simulink model "ModelloTeam1Test"  (R2022b)
settings: Solver=FixedStepAuto  StartTime=0.0  StopTime=2500  RelTol=1e-3  EnableMultiTasking=on
libraries: mbedblockslib x7
settings Model: ExtModeTrigDuration=10  Creator=giova  LastModifiedBy=giova
settings OptimizationCC: EnhancedBackFolding=on  PassReuseOutputArgsAs=Individual arguments  ZeroExternalMemoryAtStartup=off  ZeroInternalMemoryAtStartup=off  MaxStackSize=64  OptimizeBlockOrder=speed  DifferentSizesBufferReuse=on  OptimizationCustomize=off  EfficientTunableParamExpr=on
settings DebuggingCC: InheritedTsInSrcMsg=error  ParameterTunabilityLossMsg=error
settings HardwareCC: ProdBitPerPointer=32  ProdBitPerSizeT=32  ProdBitPerPtrDiffT=32  ProdLargestAtomicInteger=Long  ProdLargestAtomicFloat=Double  ProdWordSize=32  ProdLongLongMode=on  ProdHWDeviceType=ARM Compatible->ARM Cortex  UseEmbeddedCoderFeatures=off
settings SFSimCC: MATLABDynamicMemAlloc=off
settings RTWCC: Description=Embedded Coder  SystemTargetFile=ert.tlc  HardwareBoard=STM32 Nucleo F401RE  TLCOptions=-aInlineSetEventsForThisBaseRateFcn=TLC_FALSE -aSuppressMultiTaskScheduler=TLC_FALSE -aRateBasedStepFcn=1  TemplateMakefile=ert_default_tmf  Toolchain=GNU Tools for ARM Embedded Processors
settings CodeAppCC: ForceParamTrailComments=on  IgnoreCustomStorageClasses=off  OperatorAnnotations=on  SimulinkDataObjDesc=on  SFDataObjDesc=on  InsertBlockDesc=on
settings ERTTargetCC: SupportNonInlinedSFcns=on  ExtModeTransport=3  ExtModeStaticAlloc=on  ExtModeStaticAllocSize=2000  ExtModeMexFile=ext_xcp  ExtModeIntrfLevel=Level2 - Open

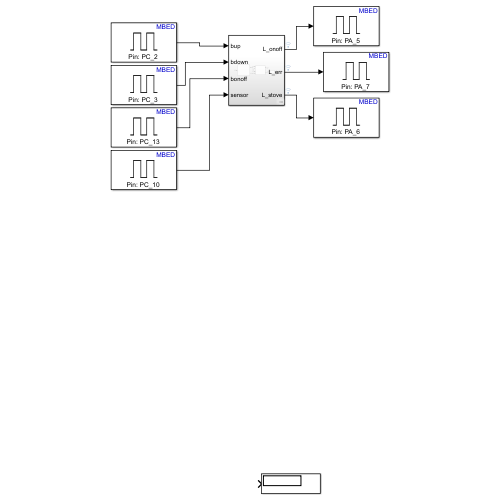
[thumbnail: Simulink's stored preview of the top-level diagram]
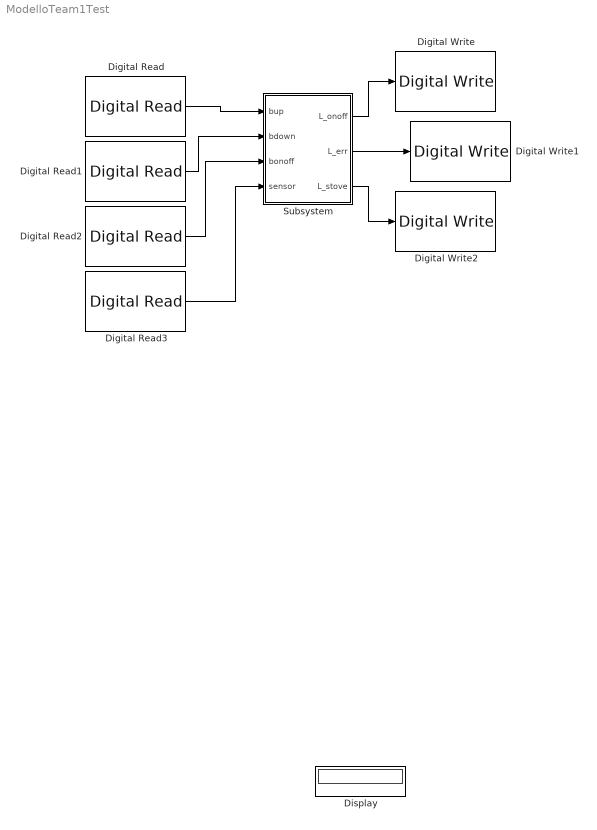
== system ModelloTeam1Test ==
  Digital Read : mbedblockslib/Digital Read  Pin=PC_2  Direction=input  SampleTime=-1
      settings: LibrarySourceBlock=stmnucleorootlib/Common/Digital Read
  Digital Read1 : mbedblockslib/Digital Read  Pin=PC_3  Direction=input  SampleTime=-1
      settings: LibrarySourceBlock=stmnucleorootlib/Common/Digital Read
  Digital Read2 : mbedblockslib/Digital Read  Pin=PC_13  Direction=input  SampleTime=-1
      settings: LibrarySourceBlock=stmnucleorootlib/Common/Digital Read
  Digital Read3 : mbedblockslib/Digital Read  Pin=PC_10  Direction=input  SampleTime=-1
      settings: LibrarySourceBlock=stmnucleorootlib/Common/Digital Read
  Digital Write : mbedblockslib/Digital Write  Pin=PA_5  Direction=output
      settings: LibrarySourceBlock=stmnucleorootlib/Common/Digital Write
  Digital Write1 : mbedblockslib/Digital Write  Pin=PA_7  Direction=output
      settings: LibrarySourceBlock=stmnucleorootlib/Common/Digital Write
  Digital Write2 : mbedblockslib/Digital Write  Pin=PA_6  Direction=output
      settings: LibrarySourceBlock=stmnucleorootlib/Common/Digital Write
  Display : Display
  Subsystem : Subsystem
  wires:
  Digital Read/1 -> Subsystem/1(bup)
  Digital Read1/1 -> Subsystem/2(bdown)
  Digital Read2/1 -> Subsystem/3(bonoff)
  Digital Read3/1 -> Subsystem/4(sensor)
  Subsystem/1(L_onoff) -> Digital Write/1
  Subsystem/2(L_err) -> Digital Write1/1
  Subsystem/3(L_stove) -> Digital Write2/1

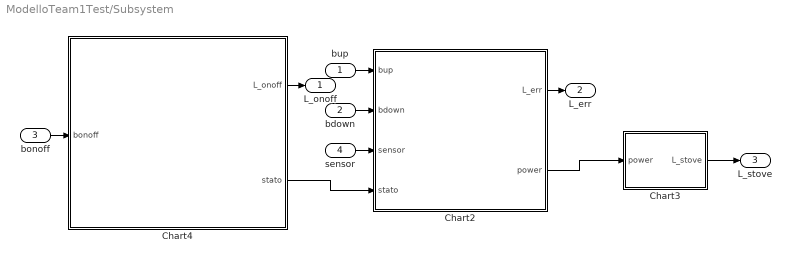
== system ModelloTeam1Test/Subsystem ==
  bup : Inport
  bdown : Inport  Port=2
  bonoff : Inport  Port=3
  sensor : Inport  Port=4
  Chart2 : Stateflow chart  TreatAsAtomicUnit=on
  Chart3 : Stateflow chart  TreatAsAtomicUnit=on
  Chart4 : Stateflow chart  TreatAsAtomicUnit=on
  L_onoff : Outport
  L_err : Outport  Port=2
  L_stove : Outport  Port=3
  wires:
  bdown/1 -> Chart2/2(bdown)
  bup/1 -> Chart2/1(bup)
  Chart2/2(power) -> Chart3/1(power)
  Chart3/1(L_stove) -> L_stove/1
  sensor/1 -> Chart2/3(sensor)
  Chart2/1(L_err) -> L_err/1
  bonoff/1 -> Chart4/1(bonoff)
  Chart4/1(L_onoff) -> L_onoff/1
  Chart4/2(stato) -> Chart2/4(stato)

== stateflow chart ModelloTeam1Test/Subsystem/Chart3 ==
  settings: updateMethod=DISCRETE  sampleTime=0.25
  state Stove_management
    state Blinking_stove
      state Led_on
        en: L_stove=ON;
      state Led_off
        en: L_stove = OFF;
      (default) -> Led_on
      Led_off -> Led_on : after(power,sec)
      Led_on -> Led_off : after(power,sec)
    state Starting_power
      en: L_stove=OFF;
    (default) -> Starting_power
    Blinking_stove -> Starting_power : [power==MAX_TIMING]
    Starting_power -> Blinking_stove : [power<MAX_TIMING]
  data: ON local =true; OFF local =false; L_stove output; power input; MAX_TIMING local =4

== stateflow chart ModelloTeam1Test/Subsystem/Chart2 ==
  settings: updateMethod=DISCRETE  sampleTime=0.25
  state Power_and_error_management
    state Power_management [parallel]
      settings: executionOrder=1
      state PowerUD_manager_on
        state PowerUp
          en: temp_power=temp_power/2
        state Check_buttons
          en: power=temp_power;
        state PowerDown
          en: temp_power=temp_power*2
        PowerUp -> Check_buttons [order 4] : [power==MAX_TIMING & sensor~=ACTIVE]{temp_power=MAX_TIMING}
        PowerUp -> Check_buttons [order 2] : after(TIMER,sec)
        Check_buttons -> PowerUp [order 1] : [power~=MIN_TIMING  & bup_second==PRESSED]
        PowerUp -> PowerUp [order 3] : [temp_power~=MIN_TIMING  & bup_second==PRESSED]
        PowerUp -> PowerDown [order 1] : [bdown_second==PRESSED]
        PowerDown -> PowerUp [order 1] : [ bup_second==PRESSED]
        (default) -> Check_buttons
        Check_buttons -> PowerDown [order 2] : [power~=MAX_TIMING & bdown_second==PRESSED]
        PowerDown -> Check_buttons [order 4] : [power==MAX_TIMING & sensor~=ACTIVE]{temp_power=MAX_TIMING}
        PowerDown -> Check_buttons [order 2] : after(TIMER,sec)
        PowerDown -> PowerDown [order 3] : [temp_power~=MAX_TIMING & bdown_second==PRESSED]
      state PowerUD_manager_off
        en: temp_power=MAX_TIMING
        power=MAX_TIMING;
      (default) -> PowerUD_manager_off
      PowerUD_manager_off -> PowerUD_manager_on : [stato==ON]
      PowerUD_manager_on -> PowerUD_manager_off : [stato==OFF]
    state Button_up_down_management [parallel]
      settings: executionOrder=2
      state Button_up_down_manager_on
        state Longpressed_DOWN_button
          en: bdown_second = RELEASED;
        state Longpressed_UP_botton
          en: bup_second = RELEASED;
        state Pressed_DOWN_button
          en: bdown_second = RELEASED;
          on after(BUTTONDURATION,sec):
          bdown_second=PRESSED;
        state Pressed_UP_botton
          en: bup_second = RELEASED;
          on after(BUTTONDURATION,sec):
          bup_second=PRESSED;
        state Wait_Up_Down_button
          en: bup_second=RELEASED;
          bdown_second=RELEASED;
        Longpressed_UP_botton -> Wait_Up_Down_button : [bup==RELEASED]
        Pressed_UP_botton -> Longpressed_UP_botton [order 2] : [bup_second==PRESSED & bup == PRESSED]
        Pressed_DOWN_button -> Longpressed_DOWN_button [order 1] : [bdown_second==PRESSED & bdown == PRESSED]
        Longpressed_DOWN_button -> Wait_Up_Down_button : [bdown==RELEASED]
        Pressed_UP_botton -> Wait_Up_Down_button [order 1] : [bup==RELEASED | sensor ~=ACTIVE]
        Pressed_DOWN_button -> Wait_Up_Down_button [order 2] : [bdown==RELEASED | sensor~=ACTIVE]
        Wait_Up_Down_button -> Pressed_UP_botton [order 2] : [bup==PRESSED & sensor==ACTIVE]
        (default) -> Wait_Up_Down_button
        Wait_Up_Down_button -> Pressed_DOWN_button [order 1] : [bdown==PRESSED & sensor==ACTIVE]
      state Button_up_down_manager_off
      Button_up_down_manager_off -> Button_up_down_manager_on : [stato==ON]
      Button_up_down_manager_on -> Button_up_down_manager_off : [stato==OFF]
      (default) -> Button_up_down_manager_off
    state Error_management [parallel]
      settings: executionOrder=3
      state Error_manager_on
        state Wait_blinking
          en: power=MAX_TIMING;
          temp_power=MAX_TIMING;
        state Check_error
        state Start_error
          en: L_err=ON;
          ex: L_err =OFF;
        (default) -> Wait_blinking
        Check_error -> Wait_blinking [order 2] : [power==MAX_TIMING]
        Wait_blinking -> Check_error : [power<MAX_TIMING]
        Start_error -> Check_error [order 1] : [sensor==ACTIVE]
        Check_error -> Start_error [order 1] : [sensor~=ACTIVE]
        Start_error -> Wait_blinking [order 2] : after(ERR_TIMER,sec)
      state Error_manager_off
        en: L_err=OFF;
      Error_manager_off -> Error_manager_on : [stato==ON]
      (default) -> Error_manager_off
      Error_manager_on -> Error_manager_off : [stato==OFF]
  (default) -> Power_and_error_management
  data: bup input; bdown input; sensor input; L_err output; RELEASED local =true; PRESSED local =false; BUTTONDURATION local =1; bup_second local; bdown_second local; ACTIVE local =0; ERR_TIMER local =10; ON local =true; OFF local =false; TIMER local =5; temp_power local; power output; stato input boolean; MAX_TIMING local =4; MIN_TIMING local =0.25

== stateflow chart ModelloTeam1Test/Subsystem/Chart4 ==
  settings: updateMethod=DISCRETE  sampleTime=0.25
  state PowerOFF_management
    state PowerOFF_manager_on
      state Pressed_OFF_button
        en: bonoff_second = RELEASED;
        on after(BUTTONDURATION,sec):
        bonoff_second=PRESSED;
      state Wait_OFF_button
        en: bonoff_second=RELEASED;
      Wait_OFF_button -> Pressed_OFF_button : [bonoff == PRESSED]
      Pressed_OFF_button -> Wait_OFF_button : [bonoff==RELEASED]
      (default) -> Wait_OFF_button
    state W_post_power_off
      en: L_onoff=OFF;
      stato=OFF;
    state PowerOFF_manager_off
      en: stato=OFF;
      L_onoff=OFF;
    state W_post_power_on
      en: stato=ON;
      L_onoff=ON;
    PowerOFF_manager_on -> W_post_power_off : [bonoff_second==PRESSED]
    W_post_power_off -> PowerOFF_manager_off : [bonoff==RELEASED]
    W_post_power_on -> PowerOFF_manager_on : [bonoff==RELEASED]
    (default) -> PowerOFF_manager_off
    PowerOFF_manager_off -> W_post_power_on : [bonoff==PRESSED]
  data: L_onoff output; bonoff input; RELEASED local =true; PRESSED local =false; bonoff_second local; ON local =true; OFF local =false; BUTTONDURATION local =1; stato output
